simulink model "Gleichstrommaschine_mit_Stromregler_und_Drezahl"  (R2022a)
settings: Solver=ode45  StartTime=0  StopTime=0.2  FixedStep=T_tast/100  RelTol=1e-9
PreLoadFcn:
  | ,try, xsg_acmc_mdl_preloadfcn(bdroot, 'LoadModel'); catch, disp(lasterr); end,
PostLoadFcn:
  | , if any(exist('dsrtsu_mdlpostloadfcn', 'file') == [2, 3, 6]), try dsrtsu_mdlpostloadfcn('Execute', bdroot); catch fprintf('Error in PostLoadFcn (dsrtsu_mdlpostloadfcn) for model "%s":\n %s\n', bdroot, lasterr); end, end,
  | ,try, xsg_acmc_mdl_postloadfcn(bdroot, 'UpdateModel', 170100); catch, disp(lasterr); end,
values from neighbouring files (symbols this model uses):
  Kp_w = J/(2 * T_sigmaw)    [Stromregler_parametern.m]
  Tm_w = 15e-3    (= 0.015)    [Stromregler_parametern.m]
  Tn_i = 4 * (T_sigmai * Tq * (T_sigmai^2 + Tq^2))/(T_sigmai + Tq)^3    [Stromregler_parametern.m]
  Tn_w = 4 * T_sigmaw    (= 0.064)    [Stromregler_parametern.m]
undefined symbols (not defined in the file or in its folder): i_max, i_soll, J, km, Kp_i, Lq, Rq, Tm_i, Ts, Ud
PreSaveFcn:
  | , if any(exist('dsmpb_private', 'file') == [2, 3, 6]), try, dsmpb_private('dsmpb_mdlclblib', 'PreSave', bdroot); catch, disp(lasterr); end, end,
CloseFcn:
  | , if any(exist('dsmpb_private', 'file') == [2, 3, 6]), try, dsmpb_private('dsmpb_mdlclblib', 'Close', bdroot); catch, disp(lasterr); end, end,
Description:
  | Standard RTI1202 template.
  | Supported Matlab version:  R2017a.
settings Model: Tag=RTI1202  DSRTSU_INTERNAL_RTI_VER=500  DSRTSU_INTERNAL_RTI_TYPE=rti1202  DSRTSU_INTERNAL_RTIFPGA=90  DSMPB_DATASERVER_ModelPortLibVersion1=8  DSMPB_DATASERVER_DataServerVersion1=6  DSMPB_DATASERVER_DataServerStreamVersion1=3  Creator=adminbochmann  LastModifiedBy=Gianluca
settings SolverCC: AlgebraicLoopSolver=TrustRegion
settings DataIOCC: ReturnWorkspaceOutputs=off
settings OptimizationCC: BlockReduction=off  OptimizeBlockIOStorage=off  BufferReuse=off  GlobalBufferReuse=off  ExpressionFolding=off  LocalBlockOutputs=off  LifeSpan=inf
settings DebuggingCC: MultiTaskRateTransMsg=warning  UnconnectedInputMsg=warning  UnconnectedOutputMsg=warning  UnconnectedLineMsg=warning  SFMachineParentedDataDiag=warning  ArithmeticOperatorsInVariantConditions=warning
settings HardwareCC: ProdBitPerPointer=32  ProdBitPerSizeT=32  ProdBitPerPtrDiffT=32  ProdLargestAtomicInteger=Integer  ProdEndianess=BigEndian  ProdWordSize=32  ProdHWDeviceType=Custom Processor->Custom  TargetIntDivRoundTo=Zero  TargetEndianess=BigEndian  TargetHWDeviceType=Custom Processor->Custom
settings SFSimCC: SimUseLocalCustomCode=off  CustomCodeUndefinedFunction=UseInterfaceOnly
settings RTWCC: Description=dSPACE DS1202 Hardware Platform  SystemTargetFile=rti1202.tlc  MakeCommand=make_rti  TemplateMakefile=rti1202.tmf  RTWUseLocalCustomCode=off
settings CodeAppCC: StateflowObjectComments=on
settings STFCustomTargetCC: ParMdlRefBuildCompliant=on  GRTInterface=off  SystemTargetFile=rti1202.tlc
settings GRTTargetCC: TargetLangStandard=C89/C90 (ANSI)  CompOptLevelCompliant=off  ConcurrentExecutionCompliant=off  CombineOutputUpdateFcns=off  MatFileLogging=off  CPPClassGenCompliant=off  UseToolchainInfoCompliant=off
settings ConfigComp: CovMetricSettings=dswe

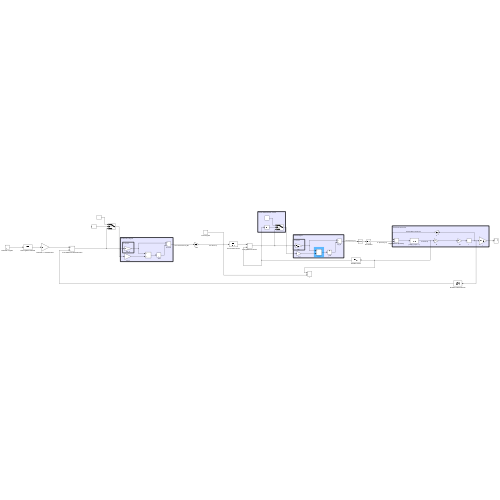
[thumbnail: Simulink's stored preview of the top-level diagram]
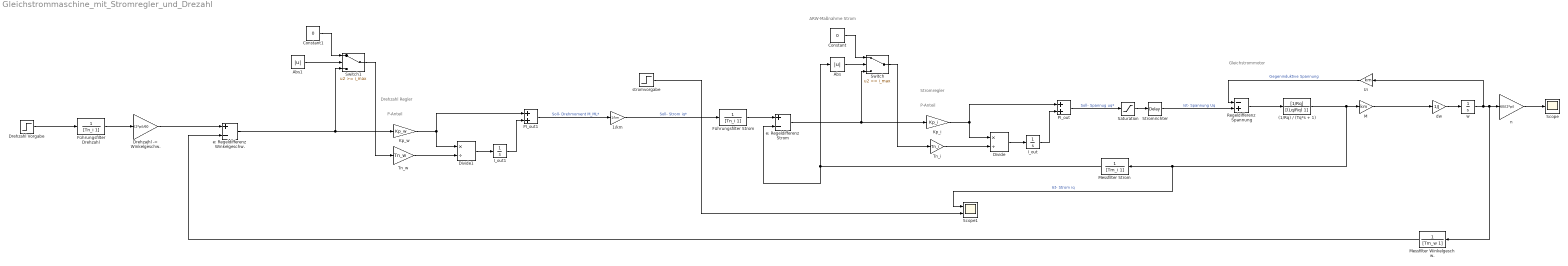
== system Gleichstrommaschine_mit_Stromregler_und_Drezahl ==
  note: Drehzahl Regler
  note: Gleichstrommotor
  note: ARW-Maßnahme Strom
  note: P-Anteil
  note: Stromregler
  note: P-Anteil
  (1/Rq) / (Tq*s + 1) : TransferFcn  Numerator=[1/Rq]  Denominator=[(Lq/Rq) 1]
  1/km : Gain  Gain=1/km
  Abs : Abs  SaturateOnIntegerOverflow=off
  Abs1 : Abs  SaturateOnIntegerOverflow=off
  Constant : Constant  Value=0
  Constant1 : Constant  Value=0
  Divide : Product  Inputs=*/
  Divide1 : Product  Inputs=*/
  Drehzahl Vorgabe : Step  Time=0.1  After=1250  SampleTime=0
  "Drehzajhl -> Winkelgeschw." : Gain  Gain=(2*pi)/60
  Führungsfilter Drehzahl : TransferFcn  Denominator=[Tn_i 1]
  Führungsfilter Strom : TransferFcn  Denominator=[Tn_i 1]
  I_out : Integrator
  I_out1 : Integrator
  Kp_i : Gain  Gain=Kp_i
  Kp_w : Gain  Gain=Kp_w
  "M " : Gain  Gain=km
  Messfilter Strom : TransferFcn  Denominator=[Tm_i 1]
  Messfilter Winkelgeschw. : TransferFcn  Denominator=[Tm_w 1]
  PI_out : Sum
  PI_out1 : Sum
  Regeldifferenz Spannung : Sum  Inputs=-+
  Saturation : Saturate  UpperLimit=Ud  LowerLimit=-Ud
  Scope : Scope
  Scope1 : Scope  NumInputPorts=2
      settings: AttributesFormatString=%<ActiveDisplayString>
  Stromrichter : TransportDelay  DelayTime=Ts/2
  Switch : Switch  Threshold=i_max  SaturateOnIntegerOverflow=off  InputSameDT=off
  Switch1 : Switch  Threshold=i_max  SaturateOnIntegerOverflow=off  InputSameDT=off
  Tn_i : Gain  Gain=Tn_i
  Tn_w : Gain  Gain=Tn_w
  Ui : Gain  Gain=km
  "dw " : Gain  Gain=1/J
  e: Regeldifferenz Strom : Sum  Inputs=+-
  e: Regeldifferenz Winkelgeschw. : Sum  Inputs=+-
  n : Gain  Gain=60/(2*pi)
  stromvorgabe : Step  Time=0.1  After=i_soll  SampleTime=0
  w : Integrator
  wires:
  "dw "/1 -> w/1
  "M "/1 -> "dw "/1
  (1/Rq) / (Tq*s + 1)/1 -> Messfilter Strom/1, Scope1/1, "M "/1  "Ist- Strom iq"
  n/1 -> Scope/1
  Saturation/1 -> Stromrichter/1
  Tn_i/1 -> Divide/2
  I_out/1 -> PI_out/2
  Divide/1 -> I_out/1
  Führungsfilter Strom/1 -> e: Regeldifferenz Strom/1
  w/1 -> Messfilter Winkelgeschw./1, n/1, Ui/1
  Regeldifferenz Spannung/1 -> (1/Rq) / (Tq*s + 1)/1
  Ui/1 -> Regeldifferenz Spannung/1  "Gegeninduktive Spannung"
  PI_out/1 -> Saturation/1  "Soll- Spannug uq*"
  e: Regeldifferenz Strom/1 -> Switch/3, Kp_i/1
  Kp_i/1 -> PI_out/1, Divide/1
  stromvorgabe/1 -> Scope1/2
  Messfilter Strom/1 -> e: Regeldifferenz Strom/2, Abs/1
  Stromrichter/1 -> Regeldifferenz Spannung/2  "Ist- Spannung Uq"
  Constant/1 -> Switch/1
  Abs/1 -> Switch/2
  Switch/1 -> Tn_i/1
  Tn_w/1 -> Divide1/2
  Divide1/1 -> I_out1/1
  Kp_w/1 -> PI_out1/1, Divide1/1
  I_out1/1 -> PI_out1/2
  Messfilter Winkelgeschw./1 -> e: Regeldifferenz Winkelgeschw./2
  e: Regeldifferenz Winkelgeschw./1 -> Switch1/3, Kp_w/1
  PI_out1/1 -> 1/km/1  "Soll- Drehmoment M_ML*"
  Drehzahl Vorgabe/1 -> Führungsfilter Drehzahl/1
  Führungsfilter Drehzahl/1 -> "Drehzajhl -> Winkelgeschw."/1
  "Drehzajhl -> Winkelgeschw."/1 -> e: Regeldifferenz Winkelgeschw./1
  Abs1/1 -> Switch1/2
  Constant1/1 -> Switch1/1
  1/km/1 -> Führungsfilter Strom/1  "Soll- Strom iq*"
  Switch1/1 -> Tn_w/1
